simulink model "battery_pack_CCCV"  (R2024b)
settings: Solver=VariableStepAuto  StartTime=0.0  StopTime=total_time  RelTol=1e-3
values from neighbouring files (symbols this model uses):
  C1 = 53958    [LoadBatteryParams.m]
  C1_pack = 53958 * (parallel/series)    (= 41592.625)    [LoadBatteryParams.m]
  C2 = 53958    [LoadBatteryParams.m]
  C2_pack = 53958 * (parallel/series)    (= 41592.625)    [LoadBatteryParams.m]
  Cc = 62.7    [LoadBatteryParams.m]
  Cs = 4.5    [LoadBatteryParams.m]
  I_CCCV_Init = I_CCCV_Init + 10    (= -690)    [GenerateCurrentProfiles.m]    (also in LoadBatteryParams.m = -400)
  Kaw = 1    [LoadBatteryParams.m]
  Ki = 50    [LoadBatteryParams.m]
  Qcell = 2.25    [LoadBatteryParams.m]
  R1 = 0.026    [LoadBatteryParams.m]
  R1_pack = 0.026 * (series/parallel)    (= 0.0337297297297)    [LoadBatteryParams.m]
  R2 = 0.026    [LoadBatteryParams.m]
  R2_pack = 0.026 * (series/parallel)    (= 0.0337297297297)    [LoadBatteryParams.m]
  Rc = 1.94    [LoadBatteryParams.m]
  Rs = 0.013    [LoadBatteryParams.m]
  Rs_pack = 0.013 * (series/parallel)    (= 0.0168648648649)    [LoadBatteryParams.m]
  Ru = 3.19    [LoadBatteryParams.m]
  SOC = OCVData(:,1)    [LoadBatteryParams.m]
  SOC_f = 0.8    [LoadBatteryParams.m]
  SOC_i = 0.2    [LoadBatteryParams.m]
  Tambient = 298    [LoadBatteryParams.m]
  TcInit = Tambient    (= 298)    [LoadBatteryParams.m]
  TsInit = Tambient    (= 298)    [LoadBatteryParams.m]
  V_des = V_des - 0.05    (= 321.13)    [GenerateCurrentProfiles.m]
  Vocv = OCVData(:,2)    [LoadBatteryParams.m]
  Vtmax_cell = 3.57    [LoadBatteryParams.m]
  Vtmin_cell = 2    [LoadBatteryParams.m]
settings Model: Creator=skylarlennon  LastModifiedBy=skylarlennon

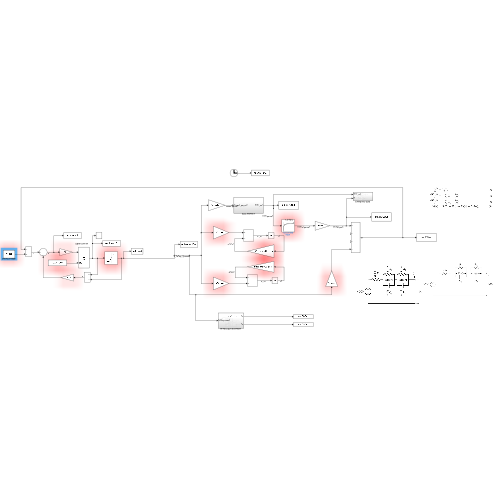
[thumbnail: Simulink's stored preview of the top-level diagram]
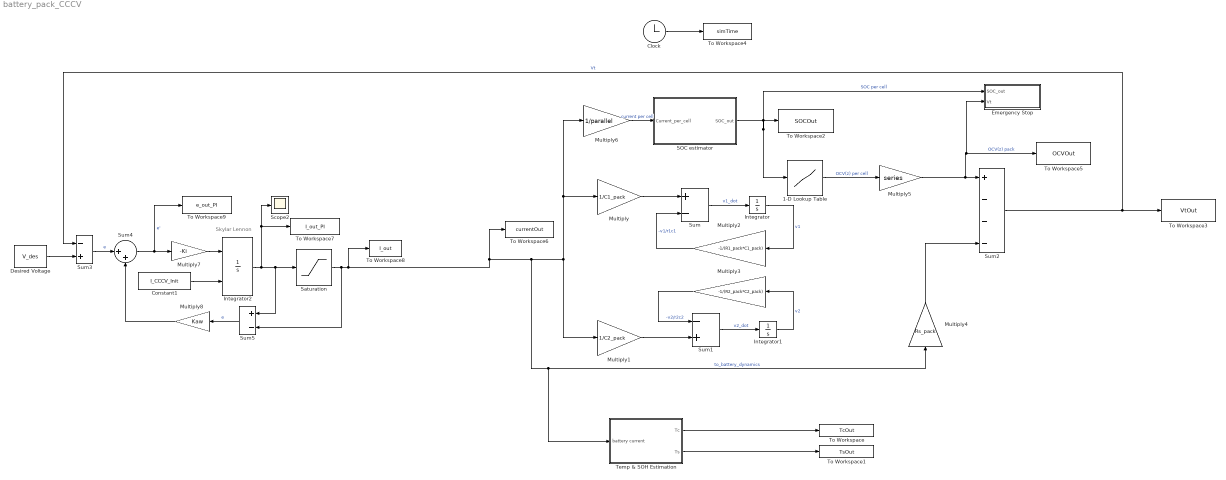
== system battery_pack_CCCV ==
  note: Skylar Lennon
  " SOC estimator" : Subsystem
  1-D Lookup Table : Lookup_n-D  NumberOfTableDimensions=1  BreakpointsForDimension1=SOC  Table=Vocv  InternalRulePriority=Speed  RndMeth=Simplest
  Clock : Clock
  Constant1 : Constant  Value=I_CCCV_Init
  Desired Voltage : Constant  Value=V_des
  Emergency Stop : Subsystem
  Integrator : Integrator
  Integrator1 : Integrator
  Integrator2 : Integrator  InitialConditionSource=external
  Multiply : Gain  Gain=1/C1_pack
  Multiply1 : Gain  Gain=1/C2_pack
  Multiply2 : Gain  Gain=-1/(R1_pack*C1_pack)
  Multiply3 : Gain  Gain=-1/(R2_pack*C2_pack)
  Multiply4 : Gain  Gain=Rs_pack
  Multiply5 : Gain  Gain=series
  Multiply6 : Gain  Gain=1/parallel
  Multiply7 : Gain  Gain=-Ki
  Multiply8 : Gain  Gain=Kaw
  Saturation : Saturate  UpperLimit=0  LowerLimit=I_CCCV_Init
  Scope2 : Scope
  Sum : Sum  Inputs=+-
  Sum1 : Sum  Inputs=-+
  Sum2 : Sum  Inputs=+---
  Sum3 : Sum  Inputs=-+
  Sum4 : Sum  Inputs=|++
  Sum5 : Sum  Inputs=+-
  Temp & SOH Estimation : Subsystem
  To Workspace : ToWorkspace  VariableName=TcOut  SampleTime=-1
  To Workspace1 : ToWorkspace  VariableName=TsOut  SampleTime=-1
  To Workspace2 : ToWorkspace  VariableName=SOCOut  SampleTime=-1
  To Workspace3 : ToWorkspace  VariableName=VtOut  SampleTime=-1
  To Workspace4 : ToWorkspace  VariableName=simTime  SampleTime=-1
  To Workspace5 : ToWorkspace  VariableName=OCVOut  SampleTime=-1
  To Workspace6 : ToWorkspace  VariableName=currentOut  SampleTime=-1
  To Workspace7 : ToWorkspace  VariableName=I_out_PI  SampleTime=-1
  To Workspace8 : ToWorkspace  VariableName=I_out  SampleTime=-1
  To Workspace9 : ToWorkspace  VariableName=e_out_PI  SampleTime=-1
  wires:
  Multiply4/1 -> Sum2/4
  Integrator/1 -> Multiply2/1  "v1"
  Clock/1 -> To Workspace4/1
  Integrator1/1 -> Multiply3/1  "v2"
  Temp & SOH Estimation/2(Ts) -> To Workspace1/1
  Multiply2/1 -> Sum/2  "-v1/r1c1"
  Multiply5/1 -> Emergency Stop/2(Vt), To Workspace5/1, Sum2/1  "OCV(z) pack"
  " SOC estimator"/1(SOC_out) -> 1-D Lookup Table/1, To Workspace2/1, Emergency Stop/1(SOC_out)  "SOC per cell"
  Multiply6/1 -> " SOC estimator"/1(Current_per_cell)  "current per cell"
  Multiply/1 -> Sum/1
  1-D Lookup Table/1 -> Multiply5/1  "OCV(z) per cell"
  Sum1/1 -> Integrator1/1  "v2_dot"
  Multiply3/1 -> Sum1/1  "-v2/r2c2"
  Multiply1/1 -> Sum1/2
  Temp & SOH Estimation/1(Tc) -> To Workspace/1
  Sum/1 -> Integrator/1  "v1_dot"
  Saturation/1 -> Sum5/2, To Workspace8/1, To Workspace6/1, Multiply1/1, Multiply/1, Multiply6/1, Temp & SOH Estimation/1(battery current), Multiply4/1  "to_battery_dynamics"
  Sum2/1 -> Sum3/1, To Workspace3/1  "Vt"
  Desired Voltage/1 -> Sum3/2
  Sum3/1 -> Sum4/1  "e"
  Integrator2/1 -> Scope2/1, To Workspace7/1, Sum5/1, Saturation/1
  Multiply7/1 -> Integrator2/1
  Sum5/1 -> Multiply8/1  "e"
  Sum4/1 -> To Workspace9/1, Multiply7/1  "e'"
  Multiply8/1 -> Sum4/2
  Constant1/1 -> Integrator2/2

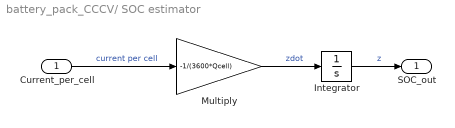
== system battery_pack_CCCV/ SOC estimator ==
  Current_per_cell : Inport
  Integrator : Integrator  InitialCondition=SOC_i
  Multiply : Gain  Gain=-1/(3600*Qcell)
  SOC_out : Outport  VectorParamsAs1DForOutWhenUnconnected=off
  wires:
  Multiply/1 -> Integrator/1  "zdot"
  Integrator/1 -> SOC_out/1  "z"
  Current_per_cell/1 -> Multiply/1  "current per cell"

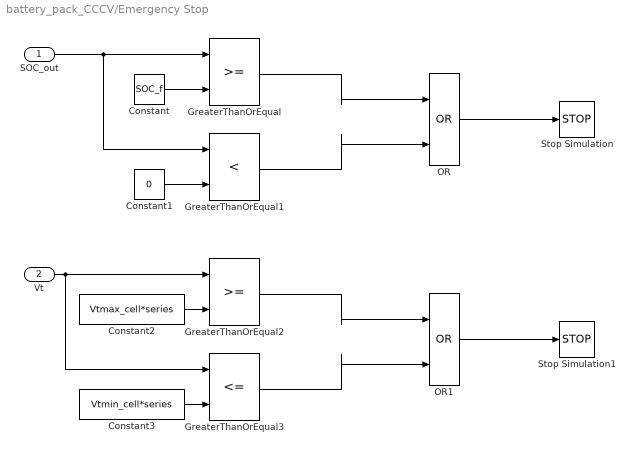
== system battery_pack_CCCV/Emergency Stop ==
  SOC_out : Inport
  Vt : Inport  Port=2
  Constant : Constant  Value=SOC_f
  Constant1 : Constant  Value=0
  Constant2 : Constant  Value=Vtmax_cell*series
  Constant3 : Constant  Value=Vtmin_cell*series
  GreaterThanOrEqual : RelationalOperator  OutDataTypeStr=boolean  RndMeth=Simplest  InputSameDT=off
  GreaterThanOrEqual1 : RelationalOperator  Operator=<  OutDataTypeStr=boolean  RndMeth=Simplest  InputSameDT=off
  GreaterThanOrEqual2 : RelationalOperator  OutDataTypeStr=boolean  RndMeth=Simplest  InputSameDT=off
  GreaterThanOrEqual3 : RelationalOperator  Operator=<=  OutDataTypeStr=boolean  RndMeth=Simplest  InputSameDT=off
  OR : Logic  Operator=OR  IconShape=distinctive  AllPortsSameDT=off  OutDataTypeStr=boolean
  OR1 : Logic  Operator=OR  IconShape=distinctive  AllPortsSameDT=off  OutDataTypeStr=boolean
  Stop Simulation : Stop
  Stop Simulation1 : Stop
  wires:
  SOC_out/1 -> GreaterThanOrEqual/1, GreaterThanOrEqual1/1
  GreaterThanOrEqual/1 -> OR/1
  OR/1 -> Stop Simulation/1
  Constant/1 -> GreaterThanOrEqual/2
  Constant1/1 -> GreaterThanOrEqual1/2
  GreaterThanOrEqual1/1 -> OR/2
  OR1/1 -> Stop Simulation1/1
  Vt/1 -> GreaterThanOrEqual2/1, GreaterThanOrEqual3/1
  Constant3/1 -> GreaterThanOrEqual3/2
  Constant2/1 -> GreaterThanOrEqual2/2
  GreaterThanOrEqual2/1 -> OR1/1
  GreaterThanOrEqual3/1 -> OR1/2

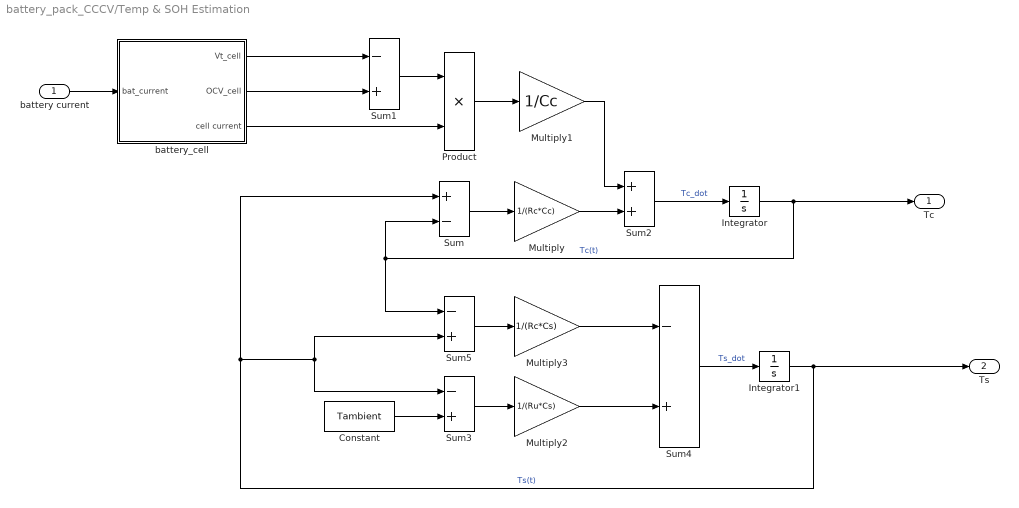
== system battery_pack_CCCV/Temp & SOH Estimation ==
  battery current : Inport
  Constant : Constant  Value=Tambient
  Integrator : Integrator  InitialCondition=TcInit
  Integrator1 : Integrator  InitialCondition=TsInit
  Multiply : Gain  Gain=1/(Rc*Cc)
  Multiply1 : Gain  Gain=1/Cc
  Multiply2 : Gain  Gain=1/(Ru*Cs)
  Multiply3 : Gain  Gain=1/(Rc*Cs)
  Product : Product
  Sum : Sum  Inputs=+-
  Sum{1,3..5} (4 alike) : Sum  Inputs=-+
  Sum2 : Sum
  battery_cell : Subsystem
  Tc : Outport
  Ts : Outport  Port=2
  wires:
  Integrator/1 -> Tc/1, Sum5/1, Sum/2  "Tc(t)"
  Sum/1 -> Multiply/1
  battery_cell/1(Vt_cell) -> Sum1/1
  battery_cell/2(OCV_cell) -> Sum1/2
  Product/1 -> Multiply1/1
  Multiply/1 -> Sum2/2
  Multiply1/1 -> Sum2/1
  Sum2/1 -> Integrator/1  "Tc_dot"
  Sum3/1 -> Multiply2/1
  Constant/1 -> Sum3/2
  Multiply2/1 -> Sum4/2
  Sum5/1 -> Multiply3/1
  Multiply3/1 -> Sum4/1
  Sum4/1 -> Integrator1/1  "Ts_dot"
  Integrator1/1 -> Ts/1, Sum/1, Sum5/2, Sum3/1  "Ts(t)"
  battery current/1 -> battery_cell/1(bat_current)
  Sum1/1 -> Product/1
  battery_cell/3(cell current) -> Product/2

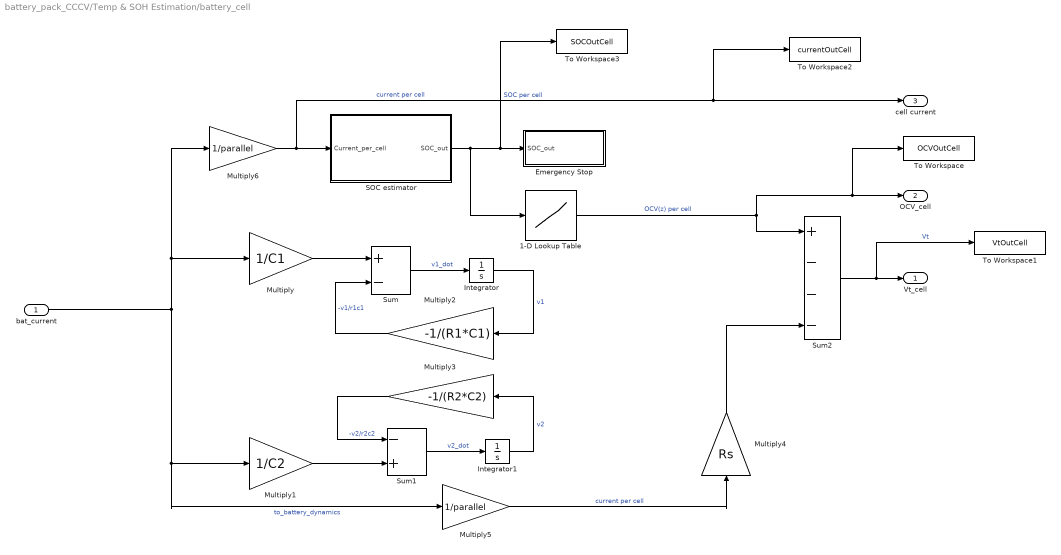
== system battery_pack_CCCV/Temp & SOH Estimation/battery_cell ==
  bat_current : Inport
  " SOC estimator" : Subsystem
  1-D Lookup Table : Lookup_n-D  NumberOfTableDimensions=1  BreakpointsForDimension1=SOC  Table=Vocv  InternalRulePriority=Speed  RndMeth=Simplest
  Emergency Stop : Subsystem
  Integrator : Integrator
  Integrator1 : Integrator
  Multiply : Gain  Gain=1/C1
  Multiply1 : Gain  Gain=1/C2
  Multiply2 : Gain  Gain=-1/(R1*C1)
  Multiply3 : Gain  Gain=-1/(R2*C2)
  Multiply4 : Gain  Gain=Rs
  Multiply5 : Gain  Gain=1/parallel
  Multiply6 : Gain  Gain=1/parallel
  Sum : Sum  Inputs=+-
  Sum1 : Sum  Inputs=-+
  Sum2 : Sum  Inputs=+---
  To Workspace : ToWorkspace  VariableName=OCVOutCell  SampleTime=-1
  To Workspace1 : ToWorkspace  VariableName=VtOutCell  SampleTime=-1
  To Workspace2 : ToWorkspace  VariableName=currentOutCell  SampleTime=-1
  To Workspace3 : ToWorkspace  VariableName=SOCOutCell  SampleTime=-1
  Vt_cell : Outport
  OCV_cell : Outport  Port=2
  cell current : Outport  Port=3
  wires:
  Multiply6/1 -> To Workspace2/1, cell current/1, " SOC estimator"/1(Current_per_cell)  "current per cell"
  Sum1/1 -> Integrator1/1  "v2_dot"
  Multiply1/1 -> Sum1/2
  Multiply3/1 -> Sum1/1  "-v2/r2c2"
  bat_current/1 -> Multiply/1, Multiply6/1, Multiply1/1, Multiply5/1  "to_battery_dynamics"
  Integrator1/1 -> Multiply3/1  "v2"
  Multiply/1 -> Sum/1
  Multiply4/1 -> Sum2/4
  Sum2/1 -> To Workspace1/1, Vt_cell/1  "Vt"
  " SOC estimator"/1(SOC_out) -> 1-D Lookup Table/1, To Workspace3/1, Emergency Stop/1(SOC_out)  "SOC per cell"
  Integrator/1 -> Multiply2/1  "v1"
  Multiply2/1 -> Sum/2  "-v1/r1c1"
  Sum/1 -> Integrator/1  "v1_dot"
  1-D Lookup Table/1 -> Sum2/1, To Workspace/1, OCV_cell/1  "OCV(z) per cell"
  Multiply5/1 -> Multiply4/1  "current per cell"

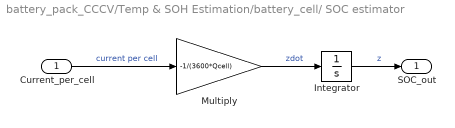
== system battery_pack_CCCV/Temp & SOH Estimation/battery_cell/ SOC estimator ==
  Current_per_cell : Inport
  Integrator : Integrator  InitialCondition=SOC_i
  Multiply : Gain  Gain=-1/(3600*Qcell)
  SOC_out : Outport  VectorParamsAs1DForOutWhenUnconnected=off
  wires:
  Multiply/1 -> Integrator/1  "zdot"
  Integrator/1 -> SOC_out/1  "z"
  Current_per_cell/1 -> Multiply/1  "current per cell"

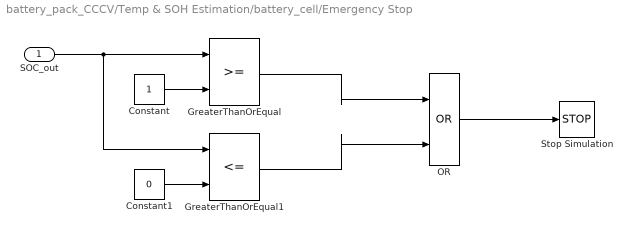
== system battery_pack_CCCV/Temp & SOH Estimation/battery_cell/Emergency Stop ==
  SOC_out : Inport
  Constant : Constant
  Constant1 : Constant  Value=0
  GreaterThanOrEqual : RelationalOperator  OutDataTypeStr=boolean  RndMeth=Simplest  InputSameDT=off
  GreaterThanOrEqual1 : RelationalOperator  Operator=<=  OutDataTypeStr=boolean  RndMeth=Simplest  InputSameDT=off
  OR : Logic  Operator=OR  IconShape=distinctive  AllPortsSameDT=off  OutDataTypeStr=boolean
  Stop Simulation : Stop
  wires:
  SOC_out/1 -> GreaterThanOrEqual/1, GreaterThanOrEqual1/1
  GreaterThanOrEqual/1 -> OR/1
  OR/1 -> Stop Simulation/1
  Constant/1 -> GreaterThanOrEqual/2
  Constant1/1 -> GreaterThanOrEqual1/2
  GreaterThanOrEqual1/1 -> OR/2
